simulink model "example_of_switch_case_subsystem"  (R2021a)
settings: Solver=VariableStepAuto  StartTime=0.0  StopTime=10.0  RelTol=1e-3
settings Model: Creator=YasserNet  LastModifiedBy=YasserNet

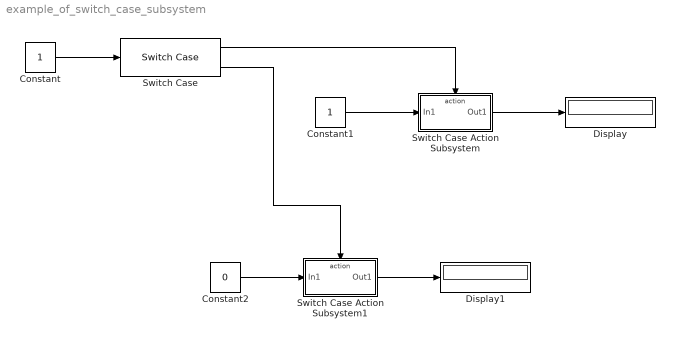
== system example_of_switch_case_subsystem ==
  Constant : Constant
  Constant1 : Constant
  Constant2 : Constant  Value=0
  Display : Display
  Display1 : Display
  Switch Case : SwitchCase
  Switch Case Action Subsystem : Subsystem  TreatAsAtomicUnit=on
  Switch Case Action Subsystem1 : Subsystem  TreatAsAtomicUnit=on
  wires:
  Constant/1 -> Switch Case/1
  Switch Case Action Subsystem/1(Out1) -> Display/1
  Switch Case/1 -> Switch Case Action Subsystem/Action
  Constant1/1 -> Switch Case Action Subsystem/1(In1)
  Constant2/1 -> Switch Case Action Subsystem1/1(In1)
  Switch Case/2 -> Switch Case Action Subsystem1/Action
  Switch Case Action Subsystem1/1(Out1) -> Display1/1

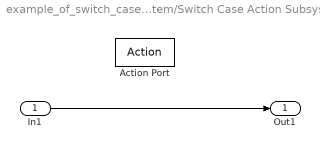
== system example_of_switch_case_subsystem/Switch Case Action Subsystem ==
  In1 : Inport
  Action Port : ActionPort  ActionPortLabel=case [ 1 ]:
  Out1 : Outport
  wires:
  In1/1 -> Out1/1

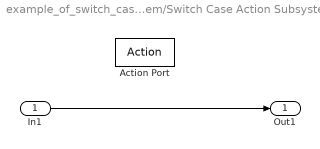
== system example_of_switch_case_subsystem/Switch Case Action Subsystem1 ==
  In1 : Inport
  Action Port : ActionPort  ActionPortLabel=default:
  Out1 : Outport
  wires:
  In1/1 -> Out1/1
